simulink model "Exercice9"  (R2024b)
settings: Solver=VariableStepAuto  StartTime=0.0  StopTime=10.0  RelTol=1e-3
settings Model: Creator=youssef bouthelja  LastModifiedBy=youssef bouthelja

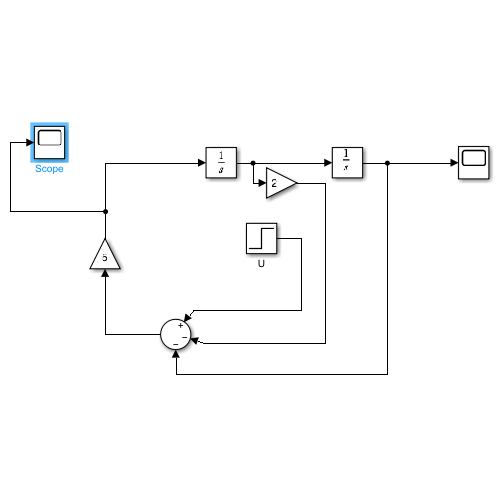
[thumbnail: Simulink's stored preview of the top-level diagram]
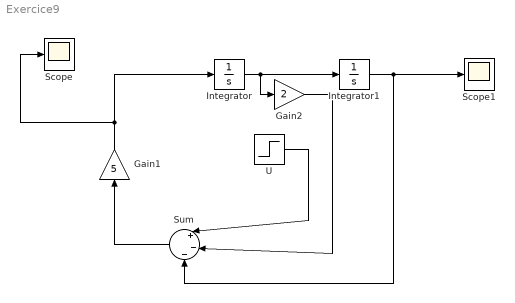
== system Exercice9 ==
  Gain1 : Gain  Gain=5
  Gain2 : Gain  Gain=2
  Integrator : Integrator
  Integrator1 : Integrator
  Scope : Scope
  Scope1 : Scope
  Sum : Sum  Inputs=|+|-|-
  U : Step  SampleTime=0
  wires:
  Gain1/1 -> Integrator/1, Scope/1
  Integrator/1 -> Integrator1/1, Gain2/1
  U/1 -> Sum/1
  Integrator1/1 -> Sum/3, Scope1/1
  Sum/1 -> Gain1/1
  Gain2/1 -> Sum/2
